simulink model "trackingAntennaOld"  (R2022b)
settings: Solver=VariableStepAuto  StartTime=0.0  StopTime=500  RelTol=1e-3
values from neighbouring files (symbols this model uses):
  J = m/12*(l^2*cos(beta)^2+d^2*sin(beta)^2+w^2)    [trackingAntennaParams.m]
  Kd = 5    [trackingAntennaParams.m]
  Kf = 0.1    [trackingAntennaParams.m]
  Kg = 2000    [trackingAntennaParams.m]
  Kt = 0.1    [trackingAntennaParams.m]
  L = 1e-5    (= 1e-05)    [trackingAntennaParams.m]
  R = 10    [trackingAntennaParams.m]
  r = 6371000    [trackingAntennaParams.m]
libraries: simulink_extras x8, sensorgpslib x1, slpidlib x1
settings Model: Creator=wenqi  LastModifiedBy=wenqi

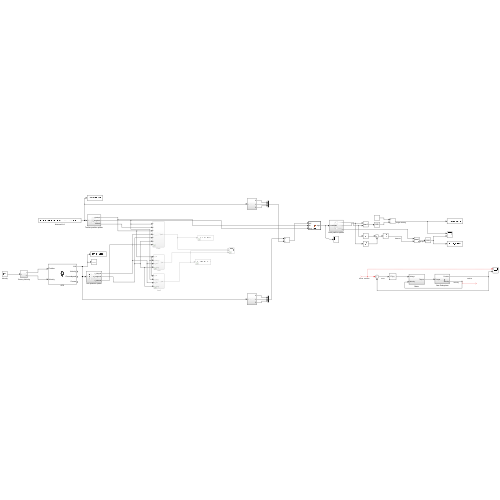
[thumbnail: Simulink's stored preview of the top-level diagram]
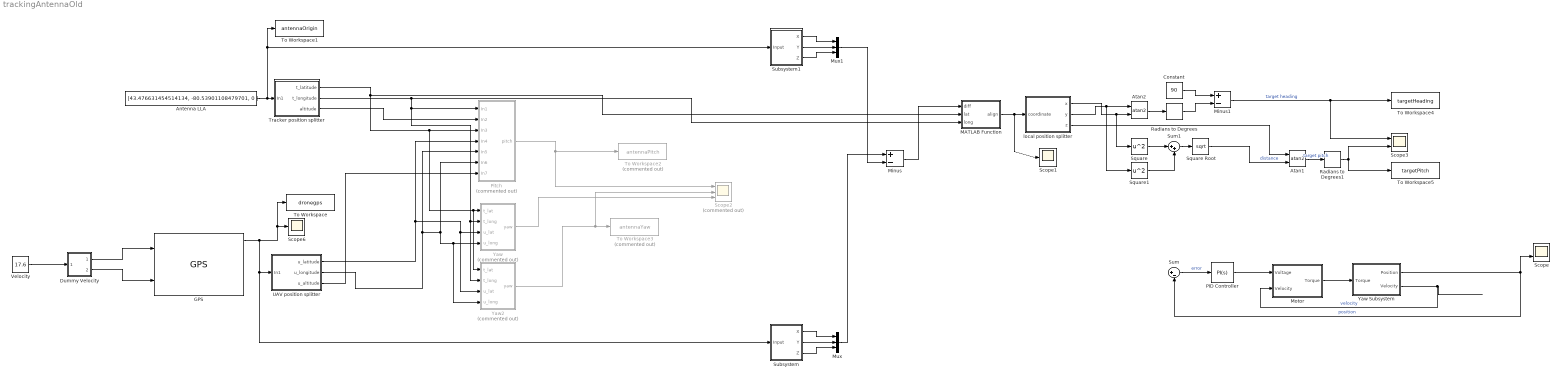
== system trackingAntennaOld ==
  Antenna LLA : Constant  Value=[43.476631454514134, -80.53901108479701, 0 ]
  Atan1 : Trigonometry  Operator=atan2
  Atan2 : Trigonometry  Operator=atan2
  Constant : Constant  Value=90
  Dummy Velocity : Subsystem
  GPS : sensorgpslib/GPS  DispRefFrame=NED  PositionInputFormat=Local  ReferenceLocation=[43.47303338903352, -80.5417882680835, 100 ]  HorizontalPositionAccuracy=1  VerticalPositionAccuracy=1  VelocityAccuracy=0.1  DecayFactor=0.999  SeedDouble=67  SimulateUsing=Interpreted execution
      settings: LibrarySourceBlock=uavsimlib/GPS
  MATLAB Function : MATLAB Function  TreatAsAtomicUnit=on
  Minus : Sum  Inputs=+-
  Minus1 : Sum  Inputs=+-
  Motor : Subsystem
  Mux : Mux  Inputs=3
  Mux1 : Mux  Inputs=3
  PID Controller : slpidlib/PID Controller  Controller=PI  Form=Parallel  TimeDomain=Continuous-time  UseExternalTs=off  SampleTime=-1  IntegratorMethod=Forward Euler  FilterMethod=Forward Euler  ControllerParametersSource=internal  P=240  I=180  UseKiTs=off  D=0  N=100  UseFilter=on  TunerSelectOption=Transfer Function Based (PID Tuner App)  InitialConditionSource=internal  InitialConditionForIntegrator=0  InitialConditionForFilter=0  DifferentiatorICPrevScaledInput=0  ExternalReset=none  TrackingMode=off  Kt=1  LimitOutput=off  SatLimitsSource=internal  UpperSaturationLimit=inf  LowerSaturationLimit=-inf  LinearizeAsGain=on  AntiWindupMode=none  Kb=1  LimitIntegrator=off  UpperIntegratorSaturationLimit=inf  LowerIntegratorSaturationLimit=-inf  POutMin=[]  POutMax=[]  IOutMin=[]  IOutMax=[]  DOutMin=[]  DOutMax=[]  NOutMin=[]  NOutMax=[]  SumOutMin=[]  SumOutMax=[]  SaturationOutMin=[]  SaturationOutMax=[]  PParamMin=[]  PParamMax=[]  IParamMin=[]  IParamMax=[]  DParamMin=[]  DParamMax=[]  NParamMin=[]  NParamMax=[]  KbParamMin=[]  KbParamMax=[]  KtParamMin=[]  KtParamMax=[]  KbOutMin=[]  KbOutMax=[]  KtOutMin=[]  KtOutMax=[]  IntegratorOutMin=[]  IntegratorOutMax=[]  FilterOutMin=[]  FilterOutMax=[]  SumI1OutMin=[]  SumI1OutMax=[]  SumI2OutMin=[]  SumI2OutMax=[]  SumI3OutMin=[]  SumI3OutMax=[]  SumI4OutMin=[]  SumI4OutMax=[]  SumDOutMin=[]  SumDOutMax=[]  DifferentiatorOutMin=[]  DifferentiatorOutMax=[]  FilterDiffOutCoefMin=[]  FilterDiffOutCoefMax=[]  ReciprocalOutMin=[]  ReciprocalOutMax=[]  SumDenOutMin=[]  SumDenOutMax=[]  SumNumOutMin=[]  SumNumOutMax=[]  DivideOutMin=[]  DivideOutMax=[]  UdiffTsProdOutMin=[]  UdiffTsProdOutMax=[]  NTsProdOutMin=[]  NTsProdOutMax=[]  UintegralTsProdOutMin=[]  UintegralTsProdOutMax=[]  UngainTsProdOutMin=[]  UngainTsProdOutMax=[]  ClampingZeroOutDataTypeStr=Inherit: Inherit via back propagation  ClampingZeroOutMin=[]  ClampingZeroOutMax=[]  FilterDenConstantOutDataTypeStr=Inherit: Inherit via back propagation  FilterDenConstantOutMin=[]  FilterDenConstantOutMax=[]  PCopyOutDataTypeStr=Inherit: Inherit via back propagation  PCopyOutMin=[]  PCopyOutMax=[]  NCopyOutDataTypeStr=Inherit: Inherit via back propagation  NCopyOutMin=[]  NCopyOutMax=[]  IntegratorContinuousStateAttributes=''  IntegratorStateMustResolveToSignalObject=off  IntegratorRTWStateStorageClass=Auto  FilterContinuousStateAttributes=''  FilterStateMustResolveToSignalObject=off  FilterRTWStateStorageClass=Auto  ParallelPVariant=InternalParameters  IdealPVariant=Disabled  IVariant=InternalParameters  DVariant=Disabled  IntegratorVariant=Continuous  SatVariant=Disabled  AWVariant=Passthrough  PCopyVariant=Disabled  TRVariant=Disabled  FdbkBlocksVariant=Forward  IdealPFdbkVariant=Disabled  SatFdbkVariant=Disabled  DerivativeFilterVariant=Disabled  NVariant=Disabled  NCopyVariant=Disabled_SignalSpec  FilterICVariant=Disabled  IntegratorICVariant=InternalICs  ExternalResetVariant=Disabled  TRSumVariant=Passthrough  SumFdbkVariant=Disabled  SumVariant=Sum_PI  TsampFilterVariant=InternalTs  TsampNgainVariant=Passthrough  TsampIntegralVariant=Passthrough  ExternalSaturationOutDataTypeStr=Inherit: Same as second input
  Pitch : Subsystem  Commented=on
  Radians to Degrees : simulink_extras/Transformations/Radians to Degrees
  Radians to Degrees1 : simulink_extras/Transformations/Radians to Degrees
  Scope : Scope  NumInputPorts=2
  Scope1 : Scope
  Scope2 : Scope  Commented=on  NumInputPorts=3
  Scope3 : Scope  NumInputPorts=2
  Scope6 : Scope
  Square : Math  Operator=square
  Square Root : Sqrt
  Square1 : Math  Operator=square
  Subsystem : Subsystem
  Subsystem1 : Subsystem
  Sum : Sum  Inputs=|+-
  Sum1 : Sum  Inputs=|++
  To Workspace : ToWorkspace  VariableName=dronegps  SaveFormat=Timeseries  SampleTime=-1
  To Workspace1 : ToWorkspace  VariableName=antennaOrigin  SaveFormat=Timeseries  SampleTime=-1
  To Workspace2 : ToWorkspace  Commented=on  VariableName=antennaPitch  SaveFormat=Timeseries  SampleTime=-1
  To Workspace3 : ToWorkspace  Commented=on  VariableName=antennaYaw  SaveFormat=Timeseries  SampleTime=-1
  To Workspace4 : ToWorkspace  VariableName=targetHeading  SaveFormat=Timeseries  SampleTime=-1
  To Workspace5 : ToWorkspace  VariableName=targetPitch  SaveFormat=Timeseries  SampleTime=-1
  Tracker position splitter : Subsystem
  UAV position splitter : Subsystem
  Velocity : Constant  Value=17.6
  Yaw : Subsystem  Commented=on
  Yaw Subsystem : Subsystem
  Yaw2 : Subsystem  Commented=on
  local position splitter : Subsystem
  wires:
  Motor/1(Torque) -> Yaw Subsystem/1(Torque)
  Yaw Subsystem/1(Position) -> Sum/2, Scope/2  "position"
  Yaw Subsystem/2(Velocity) -> Motor/2(Velocity)  "velocity"
  ? -> Scope/1, Sum/1  "drone_position"
  Sum/1 -> PID Controller/1  "error"
  PID Controller/1 -> Motor/1(Voltage)
  GPS/1 -> To Workspace/1, Scope6/1, Subsystem/1(Input), UAV position splitter/1(In1)
  Velocity/1 -> Dummy Velocity/1(In1)
  Dummy Velocity/1(Out1) -> GPS/1
  Dummy Velocity/2(Out2) -> GPS/2
  Antenna LLA/1 -> To Workspace1/1, Subsystem1/1(Input), Tracker position splitter/1(In1)
  Tracker position splitter/1(t_latitude) -> MATLAB Function/2(lat), Yaw2/1(t_lat), Yaw/1(t_lat), Pitch/3(In3)
  Tracker position splitter/2(t_longitude) -> MATLAB Function/3(long), Pitch/1(In1), Yaw2/2(t_long), Yaw/2(t_long)
  UAV position splitter/1(u_latitude) -> Pitch/4(In4), Yaw/3(u_lat), Yaw2/3(u_lat)
  UAV position splitter/2(u_longitude) -> Pitch/5(In5), Pitch/6(In6), Yaw/4(u_long), Yaw2/4(u_long)
  Tracker position splitter/3(altitude) -> Pitch/2(In2)
  UAV position splitter/3(u_altitude) -> Pitch/7(In7)
  Pitch/1(pitch) -> To Workspace2/1, Scope2/1
  Yaw2/1(yaw) -> Scope2/2, To Workspace3/1
  Yaw/1(yaw) -> Scope2/3
  Subsystem/1(X) -> Mux/1
  Subsystem/3(Z) -> Mux/3
  Subsystem/2(Y) -> Mux/2
  Mux/1 -> Minus/1
  Subsystem1/1(X) -> Mux1/1
  Subsystem1/2(Y) -> Mux1/2
  Subsystem1/3(Z) -> Mux1/3
  Mux1/1 -> Minus/2
  Minus/1 -> MATLAB Function/1(diff)
  MATLAB Function/1(align) -> Scope1/1, local position splitter/1(coordinate)
  local position splitter/2(y) -> Square1/1, Atan2/1
  local position splitter/1(x) -> Square/1, Atan2/2
  Atan2/1 -> Radians to Degrees/1
  Constant/1 -> Minus1/1
  Radians to Degrees/1 -> Minus1/2
  Minus1/1 -> Scope3/1, To Workspace4/1  "target heading"
  Square/1 -> Sum1/1
  Square1/1 -> Sum1/2
  Sum1/1 -> Square Root/1
  Square Root/1 -> Atan1/2  "distance"
  local position splitter/3(z) -> Atan1/1
  Atan1/1 -> Radians to Degrees1/1  "target pitch"
  Radians to Degrees1/1 -> Scope3/2, To Workspace5/1

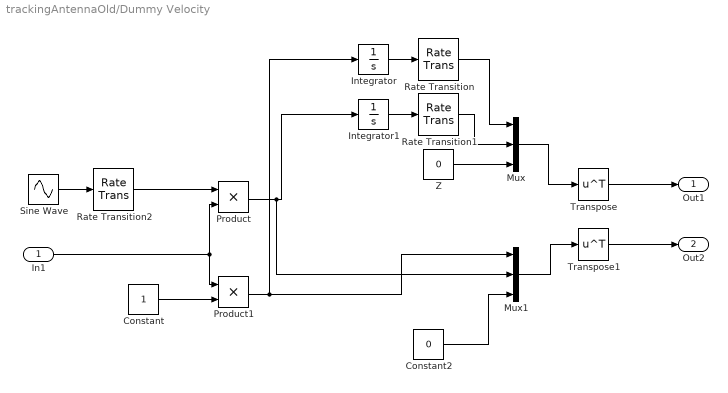
== system trackingAntennaOld/Dummy Velocity ==
  In1 : Inport
  Constant : Constant
  Constant2 : Constant  Value=0
  Integrator : Integrator
  Integrator1 : Integrator
  Mux : Mux  Inputs=3
  Mux1 : Mux  Inputs=3
  Product : Product
  Product1 : Product
  Rate Transition : RateTransition  OutPortSampleTime=1/60
  Rate Transition1 : RateTransition  OutPortSampleTime=1/60
  Rate Transition2 : RateTransition  OutPortSampleTime=1/60
  Sine Wave : Sin  Frequency=200/1800  SampleTime=0
  Transpose : Math  Operator=transpose
  Transpose1 : Math  Operator=transpose
  Z : Constant  Value=0
  Out1 : Outport
  Out2 : Outport  Port=2
  wires:
  Z/1 -> Mux/3
  Rate Transition/1 -> Mux/1
  Transpose1/1 -> Out2/1
  Transpose/1 -> Out1/1
  Constant2/1 -> Mux1/3
  In1/1 -> Product1/1, Product/2
  Integrator/1 -> Rate Transition/1
  Mux1/1 -> Transpose1/1
  Mux/1 -> Transpose/1
  Integrator1/1 -> Rate Transition1/1
  Sine Wave/1 -> Rate Transition2/1
  Product/1 -> Mux1/2, Integrator1/1
  Rate Transition1/1 -> Mux/2
  Rate Transition2/1 -> Product/1
  Constant/1 -> Product1/2
  Product1/1 -> Integrator/1, Mux1/1

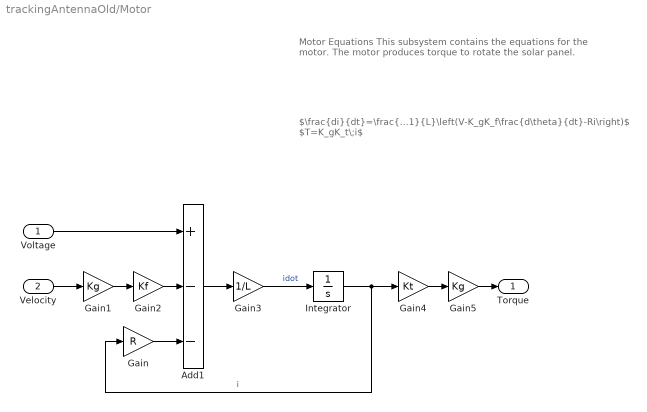
== system trackingAntennaOld/Motor ==
  note: $\frac{di}{dt}=\frac{1}{L}\left(V-K_gK_f\frac{d\theta}{dt}-Ri\right)$
      | $T=K_gK_t\;i$
  note: Motor Equations
      |
      | This subsystem contains the equations for the motor. The motor produces torque to rotate the solar panel.
  Voltage : Inport
  Velocity : Inport  Port=2
  Add1 : Sum  Inputs=+--
  Gain : Gain  Gain=R
  Gain1 : Gain  Gain=Kg
  Gain2 : Gain  Gain=Kf
  Gain3 : Gain  Gain=1/L
  Gain4 : Gain  Gain=Kt
  Gain5 : Gain  Gain=Kg
  Integrator : Integrator
  Torque : Outport
  wires:
  Voltage/1 -> Add1/1
  Gain2/1 -> Add1/2
  Gain3/1 -> Integrator/1  "idot"
  Gain/1 -> Add1/3
  Integrator/1 -> Gain4/1, Gain/1  "i"
  Add1/1 -> Gain3/1
  Velocity/1 -> Gain1/1
  Gain4/1 -> Gain5/1
  Gain1/1 -> Gain2/1
  Gain5/1 -> Torque/1

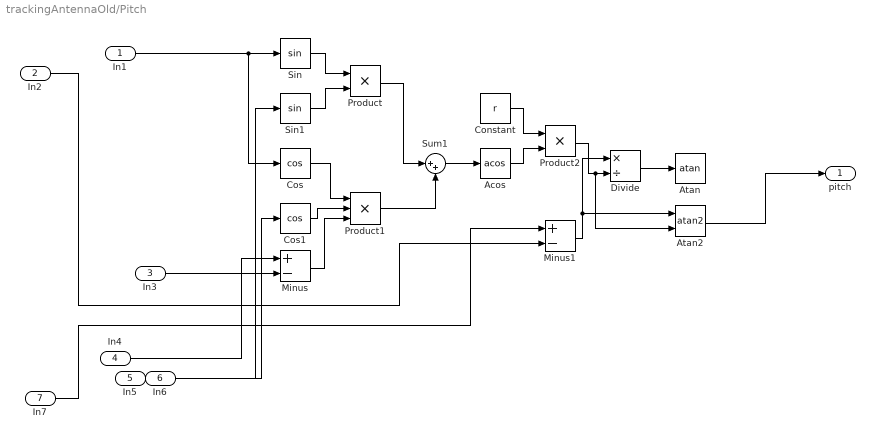
== system trackingAntennaOld/Pitch ==
  In1 : Inport
  In2 : Inport  Port=2
  In3 : Inport  Port=3
  In4 : Inport  Port=4
  In5 : Inport  Port=5
  In6 : Inport  Port=6
  In7 : Inport  Port=7
  Acos : Trigonometry  Operator=acos
  Atan : Trigonometry  Operator=atan
  Atan2 : Trigonometry  Operator=atan2
  Constant : Constant  Value=r
  Cos : Trigonometry  Operator=cos
  Cos1 : Trigonometry  Operator=cos
  Divide : Product  Inputs=*/
  Minus : Sum  Inputs=+-
  Minus1 : Sum  Inputs=+-
  Product : Product
  Product1 : Product  Inputs=3
  Product2 : Product
  Sin : Trigonometry
  Sin1 : Trigonometry
  Sum1 : Sum  Inputs=|++
  pitch : Outport
  wires:
  Product1/1 -> Sum1/2
  In1/1 -> Cos/1, Sin/1
  Cos/1 -> Product1/1
  Constant/1 -> Product2/1
  Acos/1 -> Product2/2
  Minus1/1 -> Divide/1, Atan2/1
  Minus/1 -> Product1/3
  Divide/1 -> Atan/1
  Product2/1 -> Atan2/2, Divide/2
  In3/1 -> Minus/2
  Product/1 -> Sum1/1
  Sin/1 -> Product/1
  Sin1/1 -> Product/2
  Cos1/1 -> Product1/2
  Sum1/1 -> Acos/1
  In4/1 -> Minus/1
  In6/1 -> Sin1/1
  In2/1 -> Minus1/2
  In5/1 -> Cos1/1
  In7/1 -> Minus1/1
  Atan2/1 -> pitch/1

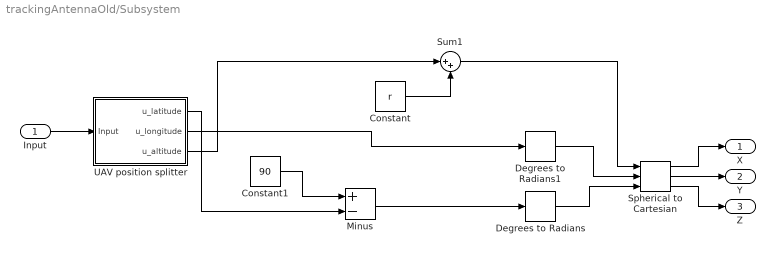
== system trackingAntennaOld/Subsystem ==
  Input : Inport
  Constant : Constant  Value=r
  Constant1 : Constant  Value=90
  Degrees to Radians : simulink_extras/Transformations/Degrees to Radians
  Degrees to Radians1 : simulink_extras/Transformations/Degrees to Radians
  Minus : Sum  Inputs=+-
  Spherical to Cartesian : simulink_extras/Transformations/Spherical to Cartesian
  Sum1 : Sum  Inputs=|++
  UAV position splitter : Subsystem
  X : Outport
  Y : Outport  Port=2
  Z : Outport  Port=3
  wires:
  Constant1/1 -> Minus/1
  Spherical to Cartesian/3 -> Z/1
  UAV position splitter/3(u_altitude) -> Sum1/1
  Spherical to Cartesian/1 -> X/1
  UAV position splitter/1(u_latitude) -> Minus/2
  Constant/1 -> Sum1/2
  Spherical to Cartesian/2 -> Y/1
  Minus/1 -> Degrees to Radians/1
  UAV position splitter/2(u_longitude) -> Degrees to Radians1/1
  Degrees to Radians/1 -> Spherical to Cartesian/3
  Degrees to Radians1/1 -> Spherical to Cartesian/2
  Sum1/1 -> Spherical to Cartesian/1
  Input/1 -> UAV position splitter/1(Input)

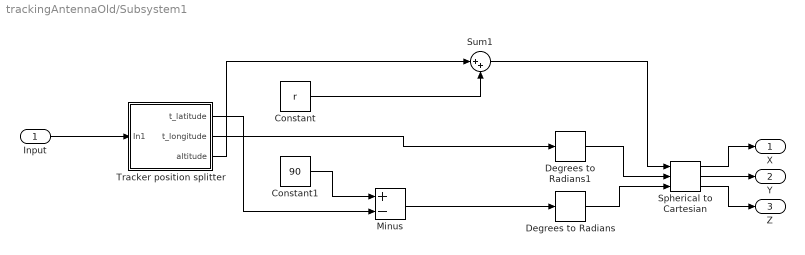
== system trackingAntennaOld/Subsystem1 ==
  Input : Inport
  Constant : Constant  Value=r
  Constant1 : Constant  Value=90
  Degrees to Radians : simulink_extras/Transformations/Degrees to Radians
  Degrees to Radians1 : simulink_extras/Transformations/Degrees to Radians
  Minus : Sum  Inputs=+-
  Spherical to Cartesian : simulink_extras/Transformations/Spherical to Cartesian
  Sum1 : Sum  Inputs=|++
  Tracker position splitter : Subsystem
  X : Outport
  Y : Outport  Port=2
  Z : Outport  Port=3
  wires:
  Constant1/1 -> Minus/1
  Spherical to Cartesian/3 -> Z/1
  Spherical to Cartesian/1 -> X/1
  Constant/1 -> Sum1/2
  Spherical to Cartesian/2 -> Y/1
  Minus/1 -> Degrees to Radians/1
  Degrees to Radians/1 -> Spherical to Cartesian/3
  Degrees to Radians1/1 -> Spherical to Cartesian/2
  Sum1/1 -> Spherical to Cartesian/1
  Tracker position splitter/3(altitude) -> Sum1/1
  Tracker position splitter/1(t_latitude) -> Minus/2
  Tracker position splitter/2(t_longitude) -> Degrees to Radians1/1
  Input/1 -> Tracker position splitter/1(In1)

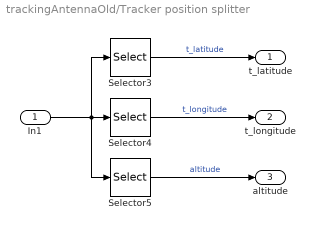
== system trackingAntennaOld/Tracker position splitter ==
  In1 : Inport
  Selector3 : Selector  InputPortWidth=3  IndexOptions=Index vector (dialog)  Indices=[1]  OutputSizes=1
  Selector4 : Selector  InputPortWidth=3  IndexOptions=Index vector (dialog)  Indices=[2]  OutputSizes=1
  Selector5 : Selector  InputPortWidth=3  IndexOptions=Index vector (dialog)  Indices=[3]  OutputSizes=1
  t_latitude : Outport
  t_longitude : Outport  Port=2
  altitude : Outport  Port=3
  wires:
  In1/1 -> Selector5/1, Selector3/1, Selector4/1
  Selector3/1 -> t_latitude/1  "t_latitude"
  Selector5/1 -> altitude/1  "altitude"
  Selector4/1 -> t_longitude/1  "t_longitude"

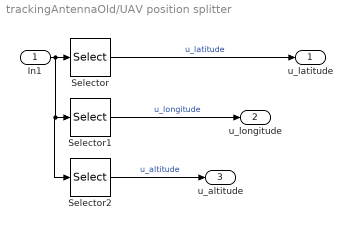
== system trackingAntennaOld/UAV position splitter ==
  In1 : Inport
  Selector : Selector  InputPortWidth=3  IndexOptions=Index vector (dialog)  Indices=[1]  OutputSizes=1
  Selector1 : Selector  InputPortWidth=3  IndexOptions=Index vector (dialog)  Indices=[2]  OutputSizes=1
  Selector2 : Selector  InputPortWidth=3  IndexOptions=Index vector (dialog)  Indices=[3]  OutputSizes=1
  u_latitude : Outport
  u_longitude : Outport  Port=2
  u_altitude : Outport  Port=3
  wires:
  In1/1 -> Selector2/1, Selector1/1, Selector/1
  Selector2/1 -> u_altitude/1  "u_altitude"
  Selector/1 -> u_latitude/1  "u_latitude"
  Selector1/1 -> u_longitude/1  "u_longitude"

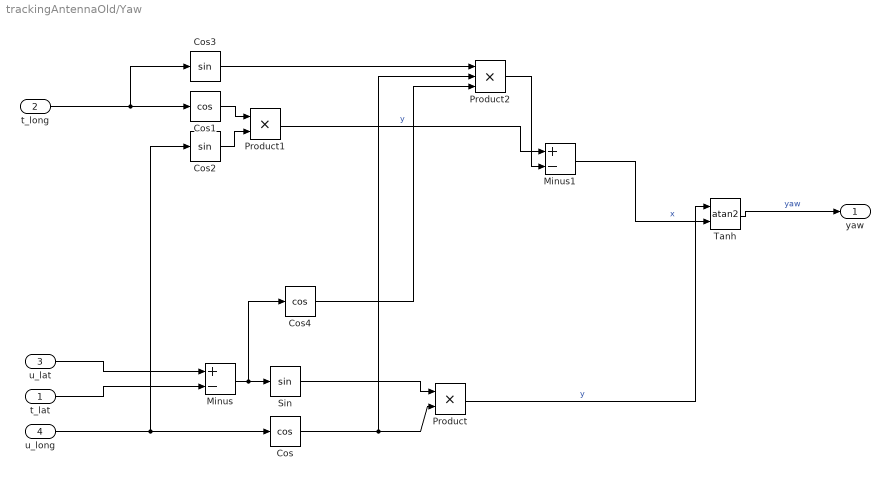
== system trackingAntennaOld/Yaw ==
  t_lat : Inport
  t_long : Inport  Port=2
  u_lat : Inport  Port=3
  u_long : Inport  Port=4
  Cos : Trigonometry  Operator=cos
  Cos1 : Trigonometry  Operator=cos
  Cos2 : Trigonometry
  Cos3 : Trigonometry
  Cos4 : Trigonometry  Operator=cos
  Minus : Sum  Inputs=+-
  Minus1 : Sum  Inputs=+-
  Product : Product
  Product1 : Product
  Product2 : Product  Inputs=3
  Sin : Trigonometry
  Tanh : Trigonometry  Operator=atan2
  yaw : Outport
  wires:
  Sin/1 -> Product/1
  Cos/1 -> Product/2, Product2/2
  Minus1/1 -> Tanh/2  "x"
  u_long/1 -> Cos2/1, Cos/1
  t_long/1 -> Cos3/1, Cos1/1
  u_lat/1 -> Minus/1
  t_lat/1 -> Minus/2
  Cos2/1 -> Product1/2
  Product1/1 -> Minus1/1  "y"
  Product2/1 -> Minus1/2
  Minus/1 -> Cos4/1, Sin/1
  Product/1 -> Tanh/1  "y"
  Cos1/1 -> Product1/1
  Cos3/1 -> Product2/1
  Cos4/1 -> Product2/3
  Tanh/1 -> yaw/1  "yaw"

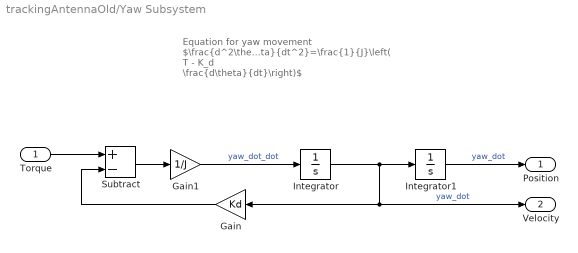
== system trackingAntennaOld/Yaw Subsystem ==
  note: Equation for yaw movement
      |
      | $\frac{d^2\theta}{dt^2}=\frac{1}{J}\left( T - K_d \frac{d\theta}{dt}\right)$
  Torque : Inport
  Gain : Gain  Gain=Kd
  Gain1 : Gain  Gain=1/J
  Integrator : Integrator
  Integrator1 : Integrator
  Subtract : Sum  Inputs=+-
  Position : Outport
  Velocity : Outport  Port=2
  wires:
  Subtract/1 -> Gain1/1
  Integrator/1 -> Velocity/1, Gain/1, Integrator1/1  "yaw_dot"
  Integrator1/1 -> Position/1  "yaw_dot"
  Gain1/1 -> Integrator/1  "yaw_dot_dot"
  Gain/1 -> Subtract/2
  Torque/1 -> Subtract/1

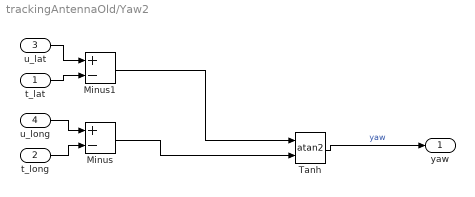
== system trackingAntennaOld/Yaw2 ==
  t_lat : Inport
  t_long : Inport  Port=2
  u_lat : Inport  Port=3
  u_long : Inport  Port=4
  Minus : Sum  Inputs=+-
  Minus1 : Sum  Inputs=+-
  Tanh : Trigonometry  Operator=atan2
  yaw : Outport
  wires:
  Tanh/1 -> yaw/1  "yaw"
  u_long/1 -> Minus/1
  t_long/1 -> Minus/2
  u_lat/1 -> Minus1/1
  t_lat/1 -> Minus1/2
  Minus1/1 -> Tanh/1
  Minus/1 -> Tanh/2

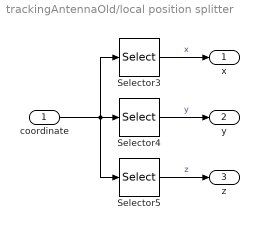
== system trackingAntennaOld/local position splitter ==
  coordinate : Inport
  Selector3 : Selector  InputPortWidth=3  IndexOptions=Index vector (dialog)  Indices=[1]  OutputSizes=1
  Selector4 : Selector  InputPortWidth=3  IndexOptions=Index vector (dialog)  Indices=[2]  OutputSizes=1
  Selector5 : Selector  InputPortWidth=3  IndexOptions=Index vector (dialog)  Indices=[3]  OutputSizes=1
  x : Outport
  y : Outport  Port=2
  z : Outport  Port=3
  wires:
  coordinate/1 -> Selector5/1, Selector3/1, Selector4/1
  Selector3/1 -> x/1  "x"
  Selector5/1 -> z/1  "z"
  Selector4/1 -> y/1  "y"

== system trackingAntennaOld/Subsystem/UAV position splitter ==
  Input : Inport
  Selector : Selector  InputPortWidth=3  IndexOptions=Index vector (dialog)  Indices=[1]  OutputSizes=1
  Selector1 : Selector  InputPortWidth=3  IndexOptions=Index vector (dialog)  Indices=[2]  OutputSizes=1
  Selector2 : Selector  InputPortWidth=3  IndexOptions=Index vector (dialog)  Indices=[3]  OutputSizes=1
  u_latitude : Outport
  u_longitude : Outport  Port=2
  u_altitude : Outport  Port=3
  wires:
  Input/1 -> Selector2/1, Selector1/1, Selector/1
  Selector2/1 -> u_altitude/1  "u_altitude"
  Selector/1 -> u_latitude/1  "u_latitude"
  Selector1/1 -> u_longitude/1  "u_longitude"

== system trackingAntennaOld/Subsystem1/Tracker position splitter ==
  In1 : Inport
  Selector3 : Selector  InputPortWidth=3  IndexOptions=Index vector (dialog)  Indices=[1]  OutputSizes=1
  Selector4 : Selector  InputPortWidth=3  IndexOptions=Index vector (dialog)  Indices=[2]  OutputSizes=1
  Selector5 : Selector  InputPortWidth=3  IndexOptions=Index vector (dialog)  Indices=[3]  OutputSizes=1
  t_latitude : Outport
  t_longitude : Outport  Port=2
  altitude : Outport  Port=3
  wires:
  In1/1 -> Selector5/1, Selector3/1, Selector4/1
  Selector3/1 -> t_latitude/1  "t_latitude"
  Selector5/1 -> altitude/1  "altitude"
  Selector4/1 -> t_longitude/1  "t_longitude"

== matlab function trackingAntennaOld/MATLAB Function ==
  data: diff input; align output; lat input; long input
function align = fcn(diff, lat, long)

    % antenna is the cartesian coordinates of the tracking antenna
    % where the origin is the center of the earth
    % z is the north pole
    % x and y are on the equator

    % diff is the cartesian coordinates of the drone relative to the
    % tracking antenna

    % want to find the difference between the drone and the antenna
    % in the antenna's local cartesian coordinates
    % where z is up, x is east, and y is north

    align = rotz(-long) * diff;
    align = roty(lat-90) * align;
    align = rotz(-90) * align;
